simulink library "Lib_HeatXfer_ThermalExpansion_org"  (Simulink 10.0)
settings: Solver=ode45  StartTime=0.0  StopTime=10.0  RelTol=1e-3  EnableMultiTasking=on
settings Model: Creator=jlkratz  LastModifiedBy=bhisma

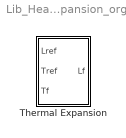
== system Lib_HeatXfer_ThermalExpansion_org ==
  Thermal Expansion : Subsystem  mask(T-MATS: Thermal Expansion Library Block){TD_M=on, alpha_M=0.000001, TVec_M=[500 1000], alphaVec_M=[0.000001 0.000001], BN_M=double(gcb)}
      mask prompts: TD_M "TD_M - Temp. dependence of the thermal expansion (unchecked - constant, checked - temp. dependent)"; alpha_M "alpha_M - Constant thermal expansion coefficient"; TVec_M "TVec_M - Temperature array (nx1)"; alphaVec_M "alphaVec_M - Thermal expansion coefficient array (alpha = f(T))(nx1)"; BN_M "Block Name"
      mask help:
      | This function calculates the length or radius of a structure that has expanded or contracted due to thermal expansion. The block accepts the previous/reference length (Lref), previous/reference temperature (Tref), and current temperature (Tf) as its inputs. The user has the option to specify a constant thermal expansion coefficient or to incorporate temperature dependence by providing data that correlates the thermal expansion coefficient with temperature.
      |
      | This block is capable of accepting various units but it is important that the units be consistent across all inputs and parameters. For details on this block, see the block help menu.
      mask init:
      | %set default parameters if they are not being used
      | if TD_M == 0
      |     TVec_M = [0 5000];
      |     alphaVec_M = [10e-6 10e-6];
      | elseif TD_M == 1
      |     alpha_M = 10e-6;
      | end
      mask Help: web(which('HeatXfer_TMATS_ThermalExpansion.html'),'-helpbrowser')
      mask Callback TD_M:
      | MSK_SEC_Enables_TMATS('TD_M',2,'dis')
      | MSK_SEC_Enables_TMATS('TD_M',[3 4],'en')

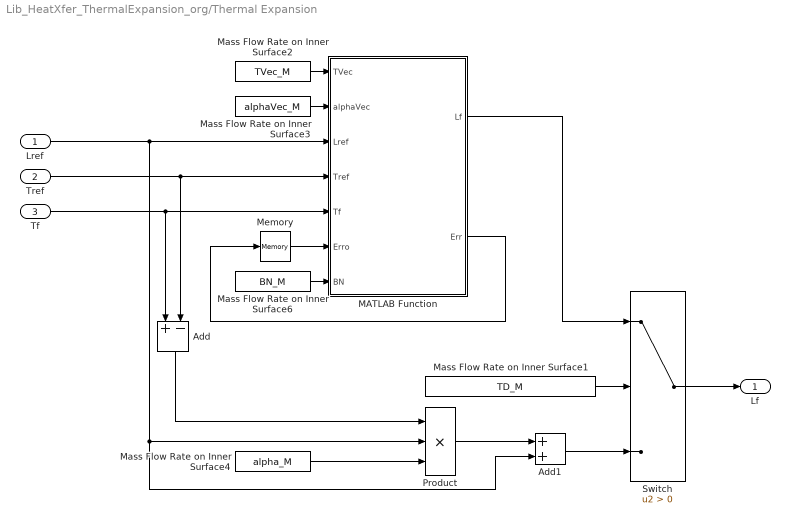
== system Lib_HeatXfer_ThermalExpansion_org/Thermal Expansion ==
  Lref : Inport
  Tref : Inport  Port=2
  Tf : Inport  Port=3
  Add : Sum  Inputs=+-
  Add1 : Sum
  MATLAB Function : MATLAB Function  TreatAsAtomicUnit=on
  Mass Flow Rate on Inner Surface1 : Constant  Value=TD_M
  Mass Flow Rate on Inner Surface2 : Constant  Value=TVec_M
  Mass Flow Rate on Inner Surface3 : Constant  Value=alphaVec_M
  Mass Flow Rate on Inner Surface4 : Constant  Value=alpha_M
  Mass Flow Rate on Inner Surface6 : Constant  Value=BN_M
  Memory : Memory  InitialCondition=zeros(1,7)
  Product : Product  Inputs=***
  Switch : Switch  Criteria=u2 > Threshold
  Lf : Outport
  wires:
  Lref/1 -> Product/2, Add1/2, MATLAB Function/3(Lref)
  Tref/1 -> MATLAB Function/4(Tref), Add/2
  Tf/1 -> MATLAB Function/5(Tf), Add/1
  Mass Flow Rate on Inner Surface6/1 -> MATLAB Function/7(BN)
  MATLAB Function/1(Lf) -> Switch/1
  Memory/1 -> MATLAB Function/6(Erro)
  MATLAB Function/2(Err) -> Memory/1
  Mass Flow Rate on Inner Surface1/1 -> Switch/2
  Mass Flow Rate on Inner Surface2/1 -> MATLAB Function/1(TVec)
  Mass Flow Rate on Inner Surface3/1 -> MATLAB Function/2(alphaVec)
  Add/1 -> Product/1
  Mass Flow Rate on Inner Surface4/1 -> Product/3
  Switch/1 -> Lf/1
  Product/1 -> Add1/1
  Add1/1 -> Switch/3

== matlab function Thermal Expansion/MATLAB Function ==
  data: TVec input double; Lf output double; alphaVec input double; Lref input double; Tref input double; Tf input double; Erro input double; BN input double; Err output double
function [Lf,Err] = ThermalExpansion(TVec,alphaVec,Lref,Tref,Tf,Erro,BN)

% initialize error/warning array
Err = Erro;
ErrNum = 1; %Error index

n = 50;

%check input sizes
if length(TVec) < 2 && Erro(ErrNum) == 0
    Err(ErrNum) = 1;
    fprintf('warning in %s: The temperature data array (T_data) must be an array of at least 2 elements\n',char(BN));
end
ErrNum = ErrNum + 1;
if length(TVec) ~= length(alphaVec) && Erro(ErrNum) == 0
    Err(ErrNum) = 1;
    fprintf('warning in %s: The temperature data array (T_data) and corresponding thermal expansion coefficient data array (alpha_data) must be the same size\n',char(BN));
end
ErrNum = ErrNum + 1;
    
%check that To and Tf are in the range of T_data
if Tref < min(TVec)
    Tref = min(TVec);
    Err(ErrNum) = 1;
    if Erro(ErrNum) == 0
        fprintf('warning in %s: The previous/reference temperature (To) is less than the minimum value of the temperature data array T_data. Expand the data arrays to assure good results. The previous/reference temperature (To) has been set to the minimum value of T_data to avoid errors.\n',char(BN));
    end
end
ErrNum = ErrNum + 1;
if Tref > max(TVec)
    Tref = max(TVec);
    Err(ErrNum) = 1;
    if Erro(ErrNum) == 0
        fprintf('warning in %s: The previous/reference temperature (To) is greater than the maximum value of the temperature data array T_data. Expand the data arrays to assure good results. The previous/reference temperature (To) has been set to the maximum value of T_data to avoid errors.\n',char(BN));
    end
end
ErrNum = ErrNum + 1;
if Tf < min(TVec)
    Tf = min(TVec);
    Err(ErrNum) = 1;
    if Erro(ErrNum) == 0
        fprintf('warning in %s: The current temperature (Tf) is less than the minimum value of the temperature data array T_data. Expand the data arrays to assure good results. The current temperature (Tf) has been set to the maximum value of T_data to avoid errors.\n',char(BN));
    end
end
ErrNum = ErrNum + 1;
if Tf > max(TVec)
    Tf = max(TVec);
    Err(ErrNum) = 1;
    if Erro(ErrNum) == 0
        fprintf('warning in %s: The current temperature (Tf) is greater than the maximum value of the temperature data array T_data. Expand the data arrays to assure good results. The current temperature (Tf) has been set to the maximum value of T_data to avoid errors.\n',char(BN));
    end
end
ErrNum = ErrNum + 1;

%check that T_data is monotonically increasing
diffT = diff(TVec);
if min(diffT) <= 0 && Erro(ErrNum) == 0
    Err(ErrNum) = 1;
    fprintf('warning in %s: The temperature data array (T_data) must be monotonically increasing\n',char(BN));
end

% Begin Calculations

Tf = linspace(Tref,Tf,n);
alpha = zeros(1,n);
for i = 1:n
    alpha(i) = interp1(TVec,alphaVec,Tf(i),'linear');
end

Int_alphadT = trapz(Tf,alpha);
dL = Lref*Int_alphadT;

Lf = Lref + dL;
